simulink model "dtc_gpc_instavel_sim"  (R2020a)
settings: Solver=VariableStepAuto  StartTime=0.0  StopTime=tsim  MaxStep=0.01  RelTol=1e-3
values from neighbouring files (symbols this model uses):
  amppert = 0    [dtc_gpc_instavel.m]
  ampref = 0.6    [dtc_gpc_instavel.m]
  Fdtc = Ftemp    [dtc_gpc_instavel.m]
  Hdtc = cell2mat(H)    [dtc_gpc_instavel.m]
  Kdtc1 = [Kdtc1; Kdtc(sum(Nu(1:i-1))+1,:)]    [dtc_gpc_instavel.m]
  tpert = 30    [dtc_gpc_instavel.m]
  tref = 5    [dtc_gpc_instavel.m]
  Ts = 1    [dtc_gpc_instavel.m]
  zr_dtc = blkdiag(zr_dtc,ones(Ny(i),1))    [dtc_gpc_instavel.m]
libraries: cstblocks x5, simulink x1
settings Model: Creator=treezao  LastModifiedBy=Usuário

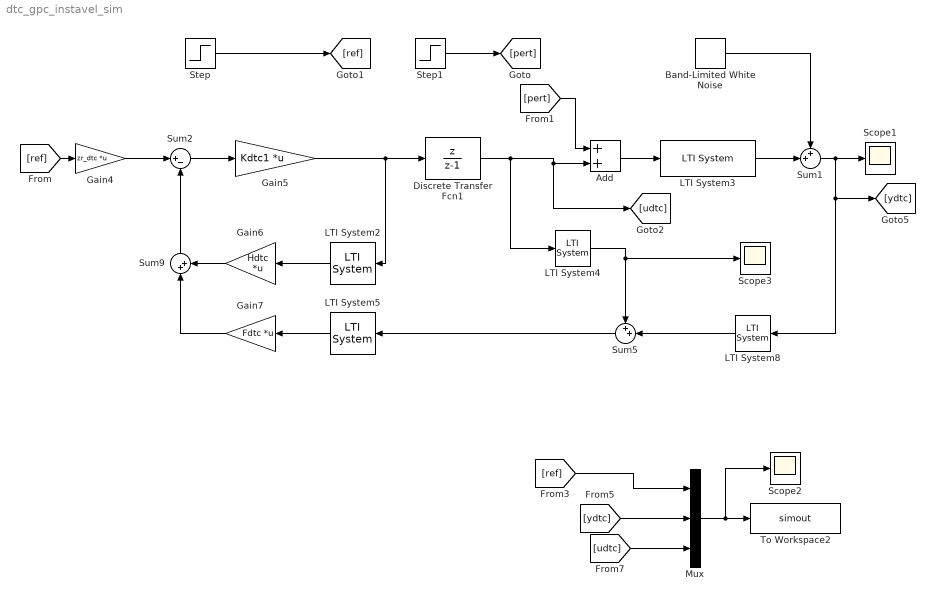
== system dtc_gpc_instavel_sim ==
  Add : Sum
  Band-Limited White Noise : simulink/Sources/Band-Limited White Noise  Cov=pRuido  Ts=Ts  seed=[23341]
  Discrete Transfer Fcn1 : DiscreteTransferFcn  Numerator=[1 0]  Denominator=[1 -1]  SampleTime=Ts
  Gain4 : Gain  Gain=zr_dtc  Multiplication=Matrix(K*u)
  Gain5 : Gain  Gain=Kdtc1  Multiplication=Matrix(K*u)
  Gain6 : Gain  Gain=Hdtc  Multiplication=Matrix(K*u)
  Gain7 : Gain  Gain=Fdtc  Multiplication=Matrix(K*u)
  LTI System2 : cstblocks/LTI System  sys=zu_dtc  IC=[]
  LTI System3 : cstblocks/LTI System  sys=P  IC=[]
  LTI System4 : cstblocks/LTI System  sys=S  IC=[]
  LTI System5 : cstblocks/LTI System  sys=zy_dtc  IC=[]
  LTI System8 : cstblocks/LTI System  sys=Fe  IC=[]
  Mux : Mux  Inputs=3
  Scope1 : Scope
  Scope2 : Scope
  Scope3 : Scope
  Step : Step  Time=tref  After=ampref  SampleTime=0
  Step1 : Step  Time=tpert  After=amppert  SampleTime=0
  Sum1 : Sum  Inputs=++|
  Sum2 : Sum  Inputs=|+-
  Sum5 : Sum  Inputs=++|
  Sum9 : Sum  Inputs=|++
  To Workspace2 : ToWorkspace  VariableName=simout  SampleTime=-1
  wires:
  Step/1 -> [ref]
  LTI System4/1 -> Sum5/1, Scope3/1
  Sum1/1 -> LTI System8/1, [ydtc], Scope1/1
  Mux/1 -> Scope2/1, To Workspace2/1
  [ref] -> Mux/1
  LTI System8/1 -> Sum5/2
  Gain6/1 -> Sum9/2
  LTI System5/1 -> Gain7/1
  LTI System2/1 -> Gain6/1
  Gain7/1 -> Sum9/1
  [ref] -> Gain4/1
  Gain5/1 -> LTI System2/1, Discrete Transfer Fcn1/1
  Gain4/1 -> Sum2/1
  Sum9/1 -> Sum2/2
  Sum2/1 -> Gain5/1
  Sum5/1 -> LTI System5/1
  Step1/1 -> [pert]
  Discrete Transfer Fcn1/1 -> Add/2, [udtc], LTI System4/1
  LTI System3/1 -> Sum1/2
  [ydtc] -> Mux/2
  [udtc] -> Mux/3
  Add/1 -> LTI System3/1
  [pert] -> Add/1
  Band-Limited White Noise/1 -> Sum1/1
